simulink model "HighPass"  (R2020a)
settings: Solver=FixedStepDiscrete  StartTime=0.0  StopTime=10.0  RelTol=1e-3
settings Model: Creator=yuzehong  LastModifiedBy=sadamu
settings OptimizationCC: DefaultParameterBehavior=Inlined  UseDivisionForNetSlopeComputation=on  GainParamInheritBuiltInType=on  UseFloatMulNetSlope=on  InlineInvariantSignals=on  OptimizeBlockIOStorage=off  BufferReuse=off  GlobalBufferReuse=off  ExpressionFolding=off  EnableMemcpy=off  PassReuseOutputArgsAs=Individual arguments  LocalBlockOutputs=off  ZeroExternalMemoryAtStartup=off  ZeroInternalMemoryAtStartup=off  NoFixptDivByZeroProtection=on  EfficientFloat2IntCast=on  LifeSpan=1  OptimizeDataStoreBuffers=off  BusAssignmentInplaceUpdate=off  OptimizationLevel=level0  OptimizationCustomize=off  EfficientTunableParamExpr=on
settings DebuggingCC: ParameterTunabilityLossMsg=error  SFMachineParentedDataDiag=error
settings HardwareCC: ProdLongLongMode=on
settings SFSimCC: MATLABDynamicMemAlloc=off  CustomCodeUndefinedFunction=UseInterfaceOnly
settings RTWCC: SystemTargetFile=ert.tlc  TemplateMakefile=ert_default_tmf
settings CodeAppCC: GenerateComments=off  IgnoreCustomStorageClasses=off  OperatorAnnotations=on  SimulinkDataObjDesc=on  SFDataObjDesc=on  CustomSymbolStrGlobalVar=rt$N$M  CustomSymbolStrType=$N$M  CustomSymbolStrFcn=$N$M$F  CustomSymbolStrMacro=$N$M  SimulinkBlockComments=off
settings ERTTargetCC: TargetLangStandard=C99 (ISO)  CodeReplacementLibrary=Intel AVX (Windows)  GenerateSampleERTMain=on  IncludeMdlTerminateFcn=off  CombineSignalStateStructs=on  SuppressErrorStatus=on  SupportAbsoluteTime=off  SupportNonFinite=off  SupportComplex=off  InlinedParameterPlacement=NonHierarchical  ERTCustomFileTemplate=example_file_process.tlc  ERTFilePackagingFormat=CompactWithDataFile

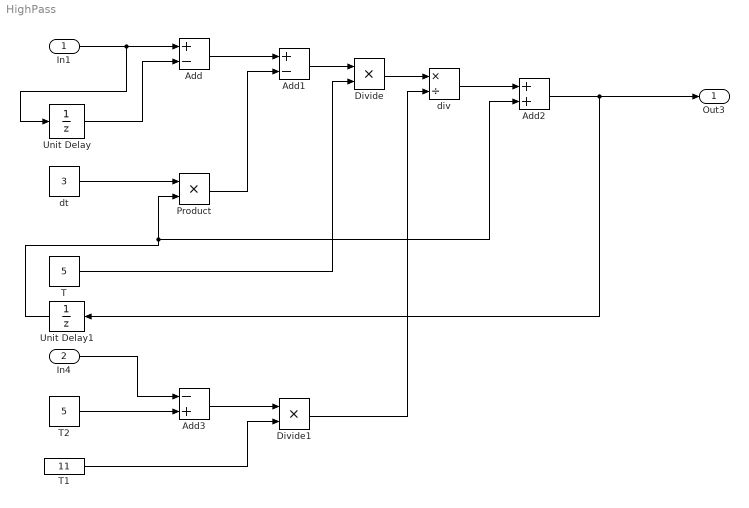
== system HighPass ==
  In1 : Inport  OutDataTypeStr=int32  PortDimensions=1
  In4 : Inport  Port=2  OutDataTypeStr=int32  PortDimensions=1
  Add : Sum  Inputs=+-
  Add1 : Sum  Inputs=+-
  Add2 : Sum
  Add3 : Sum  Inputs=-+
  Divide : Product  Inputs=**  OutDataTypeStr=int32
  Divide1 : Product  Inputs=**  OutDataTypeStr=int32  RndMeth=Simplest
  Product : Product  OutDataTypeStr=int32
  T : Constant  Value=5  OutDataTypeStr=int32  SampleTime=0.1
  T1 : Constant  Value=11  OutDataTypeStr=int32  SampleTime=0.1
  T2 : Constant  Value=5  OutDataTypeStr=int32  SampleTime=0.1
  Unit Delay : UnitDelay  SampleTime=-1  HasFrameUpgradeWarning=on
  Unit Delay1 : UnitDelay  SampleTime=-1  HasFrameUpgradeWarning=on
  div : Product  Inputs=*/  OutDataTypeStr=int32  RndMeth=Simplest
  dt : Constant  Value=3  OutDataTypeStr=int32  SampleTime=0.1
  Out3 : Outport
  wires:
  Add3/1 -> Divide1/1
  T1/1 -> Divide1/2
  Unit Delay/1 -> Add/2
  Add/1 -> Add1/1
  Divide1/1 -> div/2
  Add1/1 -> Divide/1
  dt/1 -> Product/1
  Divide/1 -> div/1
  In1/1 -> Unit Delay/1, Add/1
  T/1 -> Divide/2
  div/1 -> Add2/1
  Product/1 -> Add1/2
  Add2/1 -> Unit Delay1/1, Out3/1
  Unit Delay1/1 -> Add2/2, Product/2
  T2/1 -> Add3/2
  In4/1 -> Add3/1
